simulink model "ABS_demo212"  (R2024b)
settings: Solver=VariableStepAuto  StartTime=0.0  StopTime=10  RelTol=1e-3
undefined symbols (not defined in the file): g, I, m, R, v0
settings Model: Creator=Stephen Kingston  LastModifiedBy=bhoom
settings SolverCC: AlgebraicLoopSolver=TrustRegion
settings DebuggingCC: UnconnectedInputMsg=warning  UnconnectedOutputMsg=warning  UnconnectedLineMsg=warning
settings ModelReferenceCC: EnableRefExpFcnMdlSchedulingChecks=on
settings SFSimCC: CustomCodeUndefinedFunction=UseInterfaceOnly
settings RTWCC: GPUComputeCapability=3.5

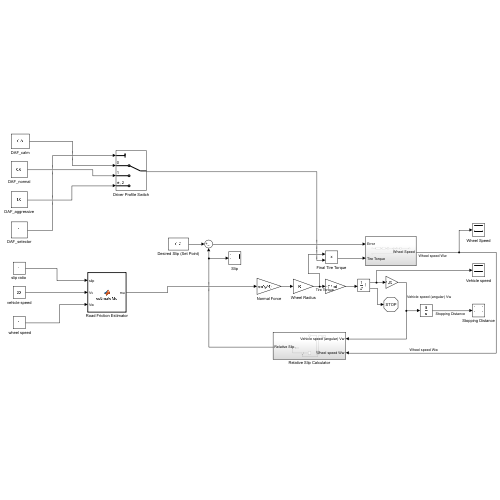
[thumbnail: Simulink's stored preview of the top-level diagram]
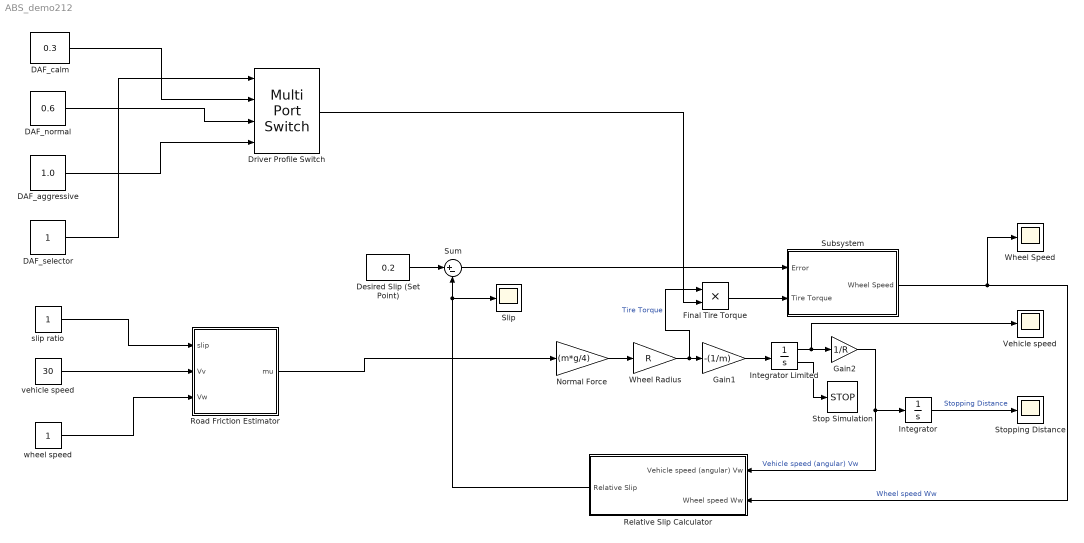
== system ABS_demo212 ==
  " wheel speed" : Constant
  DAF_aggressive : Constant  Value=1.0
  DAF_calm : Constant  Value=0.3
  DAF_normal : Constant  Value=0.6
  DAF_selector : Constant
  "Desired Slip (Set Point) " : Constant  Value=0.2
  Driver Profile Switch : MultiPortSwitch  DataPortOrder=Zero-based contiguous  zeroidx=on  SaturateOnIntegerOverflow=off  InputSameDT=off
  Final Tire Torque : Product
  Gain1 : Gain  Gain=-(1/m)
  Gain2 : Gain  Gain=1/R
  Integrator : Integrator
  Integrator Limited : Integrator  InitialCondition=v0  LimitOutput=on  UpperSaturationLimit=1000  LowerSaturationLimit=0  ShowSaturationPort=on
  Normal Force : Gain  Gain=(m*g/4)
  Relative Slip Calculator : Subsystem
  Road Friction Estimator : MATLAB Function  TreatAsAtomicUnit=on
  "Slip " : Scope
  Stop Simulation : Stop
  Stopping Distance : Scope
  Subsystem : Subsystem
  Sum : Sum  Inputs=|+-
  Vehicle speed : Scope
  Wheel Radius : Gain  Gain=R
  Wheel Speed : Scope
  "slip ratio " : Constant
  vehicle speed : Constant  Value=30
  wires:
  Sum/1 -> Subsystem/1(Error)
  Wheel Radius/1 -> Final Tire Torque/1, Gain1/1  "Tire Torque"
  Gain2/1 -> Relative Slip Calculator/1(Vehicle speed (angular) Vw), Integrator/1  "Vehicle speed (angular) Vw"
  "Desired Slip (Set Point) "/1 -> Sum/1
  Normal Force/1 -> Wheel Radius/1
  Gain1/1 -> Integrator Limited/1
  Integrator Limited/1 -> Vehicle speed/1, Gain2/1
  Integrator/1 -> Stopping Distance/1  "Stopping Distance"
  Integrator Limited/2 -> Stop Simulation/1
  Subsystem/1(Wheel Speed) -> Wheel Speed/1, Relative Slip Calculator/2(Wheel speed Ww)  "Wheel speed Ww"
  "slip ratio "/1 -> Road Friction Estimator/1(slip)
  vehicle speed/1 -> Road Friction Estimator/2(Vv)
  " wheel speed"/1 -> Road Friction Estimator/3(Vw)
  Relative Slip Calculator/1(Relative Slip) -> "Slip "/1, Sum/2
  DAF_calm/1 -> Driver Profile Switch/2
  DAF_normal/1 -> Driver Profile Switch/3
  DAF_aggressive/1 -> Driver Profile Switch/4
  DAF_selector/1 -> Driver Profile Switch/1
  Driver Profile Switch/1 -> Final Tire Torque/2
  Final Tire Torque/1 -> Subsystem/2(Tire Torque)
  Road Friction Estimator/1(mu) -> Normal Force/1

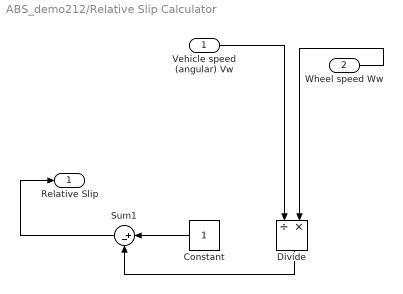
== system ABS_demo212/Relative Slip Calculator ==
  Vehicle speed (angular) Vw : Inport
  Wheel speed Ww : Inport  Port=2
  Constant : Constant
  Divide : Product  Inputs=/*
  Sum1 : Sum  Inputs=|+-
  Relative Slip : Outport  VectorParamsAs1DForOutWhenUnconnected=off
  wires:
  Divide/1 -> Sum1/2
  Sum1/1 -> Relative Slip/1
  Constant/1 -> Sum1/1
  Wheel speed Ww/1 -> Divide/2
  Vehicle speed (angular) Vw/1 -> Divide/1

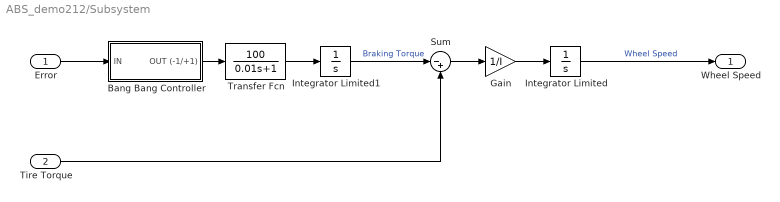
== system ABS_demo212/Subsystem ==
  Error : Inport
  Tire Torque : Inport  Port=2
  Bang Bang Controller : Subsystem
  Gain : Gain  Gain=1/I
  Integrator Limited : Integrator  InitialCondition=v0/R  LimitOutput=on  UpperSaturationLimit=1000  LowerSaturationLimit=0
  Integrator Limited1 : Integrator  LimitOutput=on  UpperSaturationLimit=1500  LowerSaturationLimit=0
  Sum : Sum  Inputs=|-+
  Transfer Fcn : TransferFcn  Numerator=[100]  Denominator=[0.01 1]
  Wheel Speed : Outport  VectorParamsAs1DForOutWhenUnconnected=off
  wires:
  Sum/1 -> Gain/1
  Transfer Fcn/1 -> Integrator Limited1/1
  Gain/1 -> Integrator Limited/1
  Integrator Limited/1 -> Wheel Speed/1  "Wheel Speed"
  Integrator Limited1/1 -> Sum/1  "Braking Torque"
  Bang Bang Controller/1(OUT (-1/+1)) -> Transfer Fcn/1
  Tire Torque/1 -> Sum/2
  Error/1 -> Bang Bang Controller/1(IN)

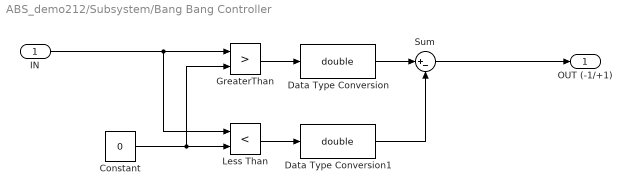
== system ABS_demo212/Subsystem/Bang Bang Controller ==
  IN : Inport
  Constant : Constant  Value=0
  Data Type Conversion : DataTypeConversion  OutDataTypeStr=double  SaturateOnIntegerOverflow=off
  Data Type Conversion1 : DataTypeConversion  OutDataTypeStr=double  SaturateOnIntegerOverflow=off
  GreaterThan : RelationalOperator  Operator=>  OutDataTypeStr=boolean  RndMeth=Simplest  InputSameDT=off
  Less Than : RelationalOperator  Operator=<  OutDataTypeStr=boolean  RndMeth=Simplest  InputSameDT=off
  Sum : Sum  Inputs=|+-
  OUT (-1/+1) : Outport  VectorParamsAs1DForOutWhenUnconnected=off
  wires:
  Sum/1 -> OUT (-1/+1)/1
  Data Type Conversion/1 -> Sum/1
  Constant/1 -> GreaterThan/2, Less Than/2
  IN/1 -> Less Than/1, GreaterThan/1
  Data Type Conversion1/1 -> Sum/2
  GreaterThan/1 -> Data Type Conversion/1
  Less Than/1 -> Data Type Conversion1/1

== matlab function ABS_demo212/Road Friction Estimator ==
  data: slip input; mu output; Vv input; Vw input
function mu = estimateMu(slip, Vv, Vw)
    % Dynamic mu-slip curve approximation
    if slip < 0.1
        mu = 10 * slip;
    elseif slip < 0.2
        mu = 1 - 10*(slip - 0.1);
    else
        mu = max(0.1, 0.6 - 3*(slip - 0.2));
    end
end
